simulink model "simulink3"  (R2016a)
settings: Solver=VariableStepAuto  StartTime=0.0  StopTime=10.0  RelTol=1e-3
settings Model: Creator=hdt04  LastModifiedBy=hdt04

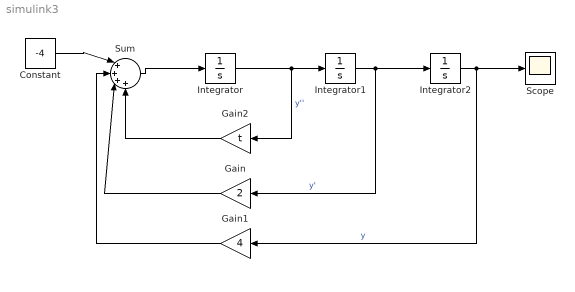
== system simulink3 ==
  Constant : Constant  Value=-4
  Gain : Gain  Gain=2
  Gain1 : Gain  Gain=4
  Gain2 : Gain  Gain=t
  Integrator : Integrator
  Integrator1 : Integrator  InitialCondition=1
  Integrator2 : Integrator  InitialCondition=1
  Scope : Scope
  Sum : Sum  Inputs=|++++
  wires:
  Integrator/1 -> Gain2/1, Integrator1/1  "y''"
  Integrator1/1 -> Gain/1, Integrator2/1  "y'"
  Integrator2/1 -> Gain1/1, Scope/1  "y"
  Constant/1 -> Sum/1
  Gain/1 -> Sum/3
  Gain1/1 -> Sum/2
  Sum/1 -> Integrator/1
  Gain2/1 -> Sum/4
